simulink model "hydraulic_test"  (R2025b)
settings: Solver=ode14x  StartTime=0.0  StopTime=2  FixedStep=1e-5  RelTol=1e-3
model workspace (MAT data in the model file):
  GateChoice = "nonlinear"
values from neighbouring files (symbols this model uses):
  k = round(i * f0 / Fs * L)    [current_test.m]
libraries: simulink x2
settings Model: Creator=LYG  LastModifiedBy=LYG

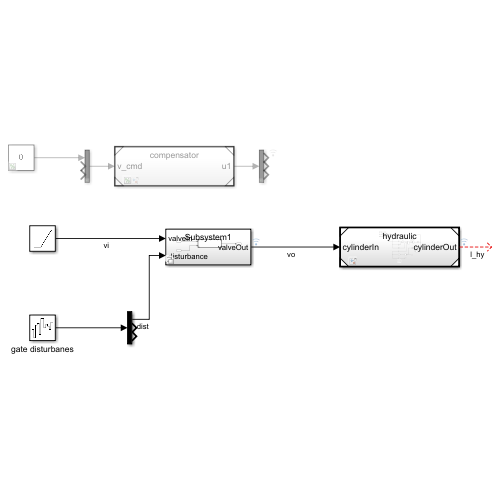
[thumbnail: Simulink's stored preview of the top-level diagram]
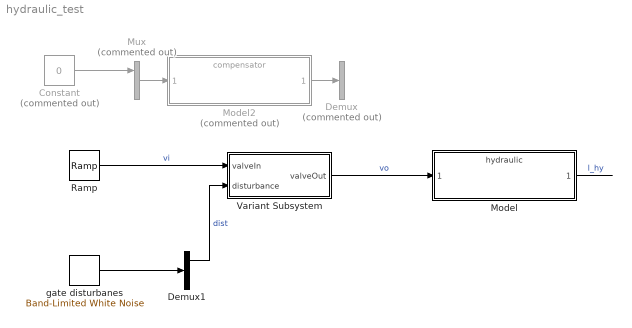
== system hydraulic_test ==
  Constant : Constant  Commented=on  Value=0
  Demux : Demux  Commented=on  Outputs=3
  Demux1 : Demux  Outputs=3
  Model : ModelReference  ModelNameDialog=hydraulic.slx  SimulationMode=Normal  ModelReferenceVersion=3.16  Ap=Ap  Ct=Ct  Fforce=Fforce  Gmass=Gmass  Kc=Kc  Kq=Kq  Ve=Ve  beta_e=beta_e  L_init=L_init
  Model2 : ModelReference  Commented=on  ModelNameDialog=compensator.slx  SimulationMode=Normal  ModelReferenceVersion=1.24
  Mux : Mux  Commented=on  Inputs=3
  Ramp : simulink/Sources/Ramp  slope=(-1 - 1) / 2  start=0  InitialOutput=1
  Variant Subsystem : Subsystem  Variant=on
  gate disturbanes : simulink/Sources/Band-Limited White Noise  Cov=2e-6 / 2  Ts=0.02  seed="[25584       50645       69937]"
  wires:
  Variant Subsystem/1(valveOut) -> Model/1  "vo"
  Mux/1 -> Model2/1
  Model2/1 -> Demux/1
  Constant/1 -> Mux/1
  Model/1 -> ?  "l_hy"
  gate disturbanes/1 -> Demux1/1
  Ramp/1 -> Variant Subsystem/1(valveIn)  "vi"
  Demux1/1 -> Variant Subsystem/2(disturbance)  "dist"

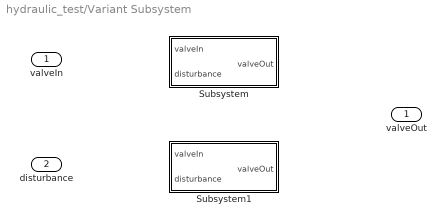
== system hydraulic_test/Variant Subsystem ==
  valveIn : Inport
  disturbance : Inport  Port=2
  Subsystem : Subsystem  VariantControl=GateChoice == 'linear'
  Subsystem1 : Subsystem  VariantControl=GateChoice == 'nonlinear'
  valveOut : Outport

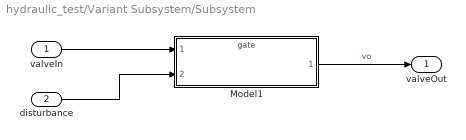
== system hydraulic_test/Variant Subsystem/Subsystem ==
  valveIn : Inport
  disturbance : Inport  Port=2
  Model1 : ModelReference  ModelNameDialog=gate.slx  SimulationMode=Normal  ModelReferenceVersion=3.12  Ksvr=Ksvr  Ksvl=Ksvl  Xmax=Xmax  Xmin=Xmin  dl=dl  dr=dr  k=k
  valveOut : Outport
  wires:
  Model1/1 -> valveOut/1  "vo"
  valveIn/1 -> Model1/1
  disturbance/1 -> Model1/2

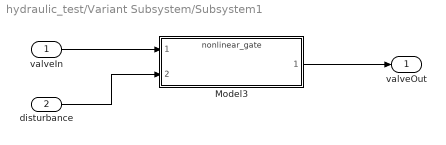
== system hydraulic_test/Variant Subsystem/Subsystem1 ==
  valveIn : Inport
  disturbance : Inport  Port=2
  Model3 : ModelReference  ModelNameDialog=nonlinear_gate.slx  SimulationMode=Normal  ModelReferenceVersion=1.18
  valveOut : Outport
  wires:
  Model3/1 -> valveOut/1
  valveIn/1 -> Model3/1
  disturbance/1 -> Model3/2
